simulink model "Navigation_Sim"  (R2023b)
settings: Solver=ode4  StartTime=0.0  StopTime=tf  FixedStep=t_step_model  RelTol=1e-3
values from neighbouring files (symbols this model uses):
  Ixx = 1    [Navigation_Script.m]    (also in Velocity_Control.m = 0.00149)
  Iyy = 1    [Navigation_Script.m]    (also in Velocity_Control.m = 0.00262)
  Izz = 1    [Navigation_Script.m]    (also in Velocity_Control.m = 0.00149)
  L = sym('L',[4 6])    [Navigation_Script.m]
  M = -1    [Navigation_Script.m]
  N = 0.9    [Navigation_Script.m]
  Q = 1.*eye(4)    [Navigation_Script.m]    (also in Velocity_Control.m = diag([1 100]))
  R = eye(6)    [Navigation_Script.m]    (also in Velocity_Control.m = eye(3))
  t_step_filter = 0.04    [Navigation_Script.m]
  t_step_model = 0.001    [Navigation_Script.m]
libraries: simulink x3
settings Model: Creator=1537565965A  LastModifiedBy=Nathan Dablain
settings SolverCC: AlgebraicLoopSolver=TrustRegion
settings OptimizationCC: DefaultUnderspecifiedDataType=single
settings DebuggingCC: UnconnectedInputMsg=warning  UnconnectedOutputMsg=warning  UnconnectedLineMsg=warning
settings ModelReferenceCC: EnableRefExpFcnMdlSchedulingChecks=on
settings SFSimCC: CustomCodeUndefinedFunction=UseInterfaceOnly

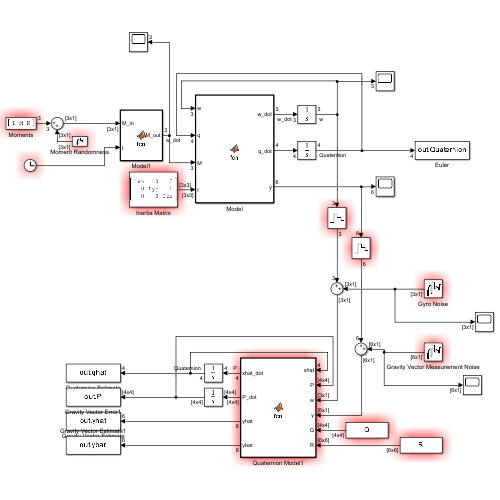
[thumbnail: Simulink's stored preview of the top-level diagram]
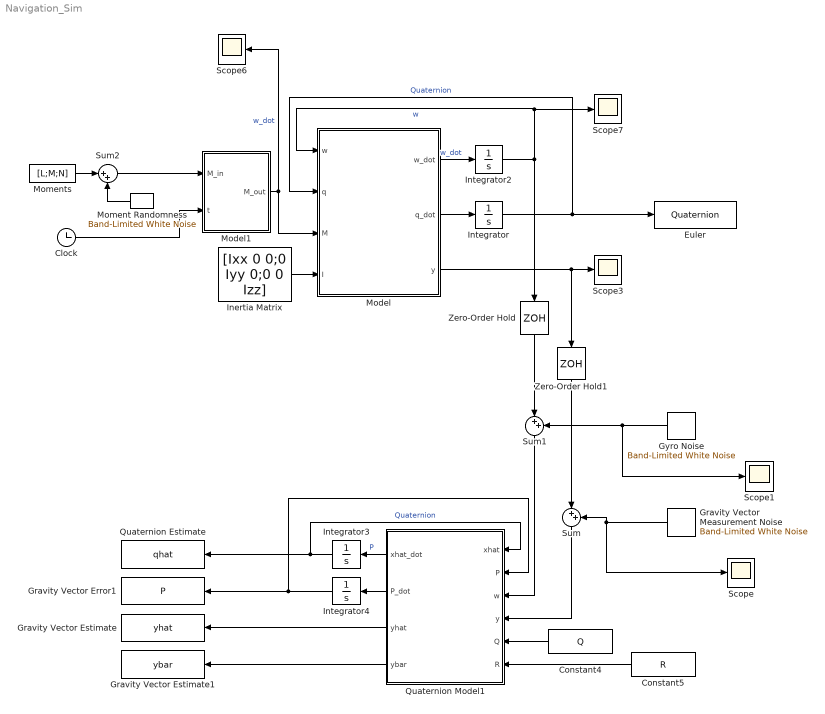
== system Navigation_Sim ==
  Clock : Clock
      settings: Decimation=1/t_step_model
  Constant4 : Constant  Value=Q
  Constant5 : Constant  Value=R
  Euler : ToWorkspace  VariableName=Quaternion  SaveFormat=Structure  SampleTime=-1
  Gravity Vector Error1 : ToWorkspace  VariableName=P  SaveFormat=Structure  SampleTime=-1
  Gravity Vector Estimate : ToWorkspace  VariableName=yhat  SaveFormat=Structure  SampleTime=-1
  Gravity Vector Estimate1 : ToWorkspace  VariableName=ybar  SaveFormat=Structure  SampleTime=-1
  Gravity Vector Measurement Noise : simulink/Sources/Band-Limited White Noise  Cov=zeros(6,1) %[.05; .05; .05; .05; .05; .05].*(t_step_model^2)  Ts=t_step_model  seed=[23341]  VectorParams1D=off
  Gyro Noise : simulink/Sources/Band-Limited White Noise  Cov=zeros(3,1) %[5; 5; 5].*(t_step_model^2)  Ts=t_step_model  seed=[23341]  VectorParams1D=off
  Inertia Matrix : Constant  Value=[Ixx 0 0;0 Iyy 0;0 0 Izz]
  Integrator : Integrator  InitialCondition=[1;0;0;0]
  Integrator2 : Integrator  InitialCondition=[0;0;0.2]
  Integrator3 : Integrator  InitialCondition=[0.7;0.1;-0.05;0.2]
  Integrator4 : Integrator  InitialCondition=zeros(4,4)
  Model : MATLAB Function  TreatAsAtomicUnit=on
  Model1 : MATLAB Function  TreatAsAtomicUnit=on
  Moment Randomness : simulink/Sources/Band-Limited White Noise  Cov=zeros(3,1)  Ts=t_step_model  seed=[23341]  VectorParams1D=off
  Moments : Constant  Value=[L;M;N]
  Quaternion Estimate : ToWorkspace  VariableName=qhat  SaveFormat=Structure  SampleTime=-1
  Quaternion Model1 : MATLAB Function  TreatAsAtomicUnit=on  SystemSampleTime=t_step_filter
  Scope{,1,3,6..7} (5 alike) : Scope
  Sum : Sum  Inputs=|++
  Sum1 : Sum  Inputs=|++
  Sum2 : Sum  Inputs=|++
  Zero-Order Hold : ZeroOrderHold  SampleTime=t_step_filter
  Zero-Order Hold1 : ZeroOrderHold  SampleTime=t_step_filter
  wires:
  Integrator/1 -> Model/2(q), Euler/1  "Quaternion"
  Model/1(w_dot) -> Integrator2/1  "w_dot"
  Integrator2/1 -> Model/1(w), Scope7/1, Zero-Order Hold/1  "w"
  Inertia Matrix/1 -> Model/4(I)
  Model/2(q_dot) -> Integrator/1
  Gravity Vector Measurement Noise/1 -> Sum/2, Scope/1
  Model/3(y) -> Scope3/1, Zero-Order Hold1/1
  Gyro Noise/1 -> Scope1/1, Sum1/2
  Quaternion Model1/3(yhat) -> Gravity Vector Estimate/1
  Moments/1 -> Sum2/1
  Moment Randomness/1 -> Sum2/2
  Model1/1(M_out) -> Scope6/1, Model/3(M)  "w_dot"
  Sum2/1 -> Model1/1(M_in)
  Clock/1 -> Model1/2(t)
  Sum1/1 -> Quaternion Model1/3(w)
  Sum/1 -> Quaternion Model1/4(y)
  Integrator4/1 -> Gravity Vector Error1/1, Quaternion Model1/2(P)
  Quaternion Model1/2(P_dot) -> Integrator4/1
  Quaternion Model1/1(xhat_dot) -> Integrator3/1  "P"
  Integrator3/1 -> Quaternion Estimate/1, Quaternion Model1/1(xhat)  "Quaternion"
  Constant4/1 -> Quaternion Model1/5(Q)
  Constant5/1 -> Quaternion Model1/6(R)
  Quaternion Model1/4(ybar) -> Gravity Vector Estimate1/1
  Zero-Order Hold1/1 -> Sum/1
  Zero-Order Hold/1 -> Sum1/1

== matlab function Navigation_Sim/Model1 ==
  data: M_in input; t input; M_out output
function M_out = fcn(M_in,t)
    if t<20
        M_out = M_in;
    else
        M_out = zeros(3,1);
    end
end

== matlab function Navigation_Sim/Model ==
  data: w input; q input; w_dot output; M input; I input; q_dot output; y output
function [w_dot,q_dot,y] = fcn(w,q,M,I)
    g = [0;0;1];
    N = [1;0;0];
    w_dot = I\(M-cross(w,I*w));
    omega = 0.5.*[0      -w(1)    -w(2)    -w(3);...
             w(1)  0       w(3)     -w(2);...
             w(2)  -w(3)   0       w(1);...
             w(3)  w(2)    -w(1)   0];
    q_dot = (omega*q)+(0.5*(1-dot(q,q))*q);
    u = q(2:4);
    t = 2*cross(u, g);
    g_rot = g + q(1)*t + cross(u, t);
    t = 2*cross(u, N);
    N_rot = N + q(1)*t + cross(u, t);
    y = [g_rot;N_rot];
    
end

== matlab function Navigation_Sim/Quaternion Model1 ==
  data: xhat input; P input; w input; xhat_dot output; y input; P_dot output; Q input; R input; yhat output; ybar output
function [xhat_dot, P_dot, yhat, ybar]  = fcn(xhat, P, w, y, Q, R)
    wx = w(1); wy = w(2); wz = w(3);
    q = xhat;

    g_vec = [0;0;1];
    t_vec = 2*cross(q(2:4), g_vec);
    g_rot = g_vec + q(1)*t_vec + cross(q(2:4), t_vec);
    n_vec = [1;0;0];
    t_vec = 2*cross(q(2:4), n_vec);
    n_rot = n_vec+q(1)*t_vec + cross(q(2:4), t_vec);
    yhat = [g_rot;n_rot];
    ybar = y-yhat;
    F = eye(4);
    H = [2*q(3)  2*q(4)  2*q(1)  2*q(2);...
        -2*q(2) -2*q(1)  2*q(4)  2*q(3);...
         0      -4*q(2) -4*q(3)  0;...
         0       0      -4*q(3) -4*q(4);...
         2*q(4)  2*q(3)  2*q(2)  2*q(1);...
        -2*q(3)  2*q(4) -2*q(1)  2*q(2)];
P = [0.9963    0.1469   -0.0064   -0.0533
    0.1469    0.6042    0.0399   -0.0111
   -0.0064    0.0399    0.3870    0.1360
   -0.0533   -0.0111    0.1360    0.5641];

    L = P*H'*inv(R);
    xhat_dot = 0.5.*[0 -wx -wy -wz;...
            wx 0 wz -wy;...
            wy -wz 0 wx;...
            wz wy -wx 0]*q + (1-dot(q,q))*q + L*ybar;
    P_dot = F*P + P*F' - L*H*P+ Q;

end
